simulink model "IcingFTISystem_simulator_rev0"  (R2021b)
settings: Solver=ode23tb  StartTime=0.0  StopTime=360  MaxStep=0.1  RelTol=1e-6
libraries: simulink x2
settings Model: Creator=julia  LastModifiedBy=julia
settings SolverCC: InitialStep=0.1

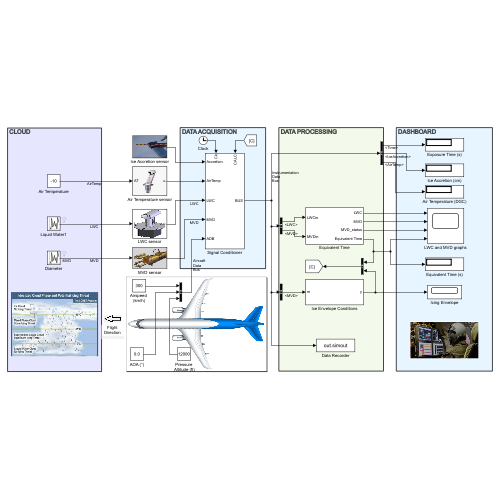
[thumbnail: Simulink's stored preview of the top-level diagram]
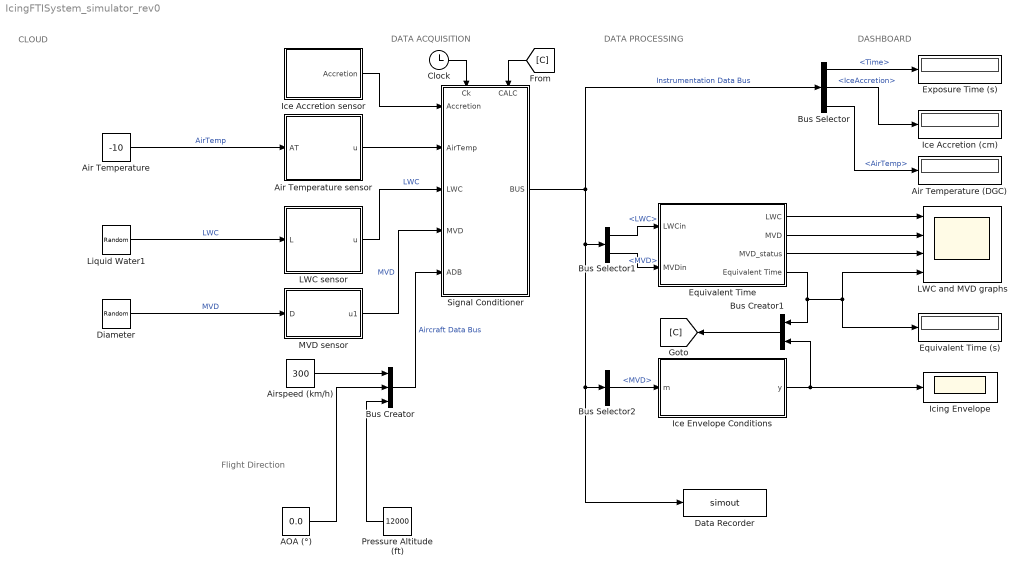
== system IcingFTISystem_simulator_rev0 ==
  note: Flight
      | Direction
  note: CLOUD
  note: DATA ACQUISITION
  note: DASHBOARD
  note: DATA PROCESSING
  AOA (°) : Constant  Value=0.0
  Air Temperature : Constant  Value=-10
  Air Temperature (DGC) : Display
  Air Temperature sensor : Subsystem
      mask Display: image('C:\Users\julia\Desktop\MEstrado\Sensores Manuais\Imagens 2022\TemperatureSensor1.jpg'); % Use "Edit Image" on toolstrip to change.
  Airspeed (km/h) : Constant  Value=300
  Bus Creator : BusCreator  Inputs=3
  Bus Creator1 : BusCreator  Inputs=2
  Bus Selector : BusSelector  OutputSignals=Time,IceAccretion,AirTemp
  Bus Selector1 : BusSelector  OutputSignals=LWC,MVD
  Bus Selector2 : BusSelector  OutputSignals=MVD
  Clock : Clock
  Data Recorder : ToWorkspace  VariableName=simout  SampleTime=1
      settings: Save2DSignal=2-D array (concatenate along first dimension)
  Diameter : UniformRandomNumber  Minimum=0  Maximum=51  SampleTime=0.5
  Equivalent Time : Subsystem
  Equivalent Time (s) : Display
  Exposure Time (s) : Display
  Ice Accretion (cm) : Display
  Ice Accretion sensor : Subsystem
      mask Display: image('C:\Users\julia\Desktop\MEstrado\Sensores Manuais\Imagens 2022\IceAccretion.jpg'); % Use "Edit Image" on toolstrip to change.
  Ice Envelope Conditions : Subsystem
  Icing Envelope : Scope
  LWC and MVD graphs : Scope  NumInputPorts=4
  LWC sensor : Subsystem
      mask Display: image('C:\Users\julia\Desktop\MEstrado\Sensores Manuais\Imagens 2022\MultielementProbe.jpg'); % Use "Edit Image" on toolstrip to change.
  Liquid Water1 : UniformRandomNumber  Minimum=0.1  Maximum=0.7  SampleTime=0.1
  MVD sensor : Subsystem
      mask Display: image('C:\Users\julia\Desktop\MEstrado\Sensores Manuais\Imagens 2022\MVDprobe.jpg'); % Use "Edit Image" on toolstrip to change.
  Pressure Altitude (ft) : Constant  Value=12000
  Signal Conditioner : Subsystem
      settings: PortSchema="{\"entries\":[{\"content\":{\"sides\":[{\"content\":{\"connectorIds\":[\"In1\",\"In2\",\"In3\",\"In4\",\"In5\"]},\"type\":\"ConnectorPlacement.EquallySpacedRectSide\",\"uuid\":\"37654887-8b06-403a-8d28-0bf4ed0ace53\"},{\"content\":{\"connectorIds\":[\"Out1\"],\"side\":\"RIGHT\"},\"type\":\"ConnectorPlacement.EquallySpacedRectSide\",\"uuid\":\"06b92d83-e4db-41b5-b404-488771456c30\"},{\"content\":{\"connectorIds\":[\"In6\",\"In7\"],\"side\":\"TOP\"},\"type\":\"ConnectorPlacement.EquallySpacedRectSide\",\"uuid\":\"374586bc-ca22-4ce3-837a-6311d85410d9\"}]},\"type\":\"ConnectorPlacement.EquallySpacedConnector\",\"uuid\":\"530a5a3a-e051-406d-b434-132ac86c67f6\"}],\"packageUris\":[\"http://schema.mathworks.com/mf0/Connector/R2020b\"],\"version\":\"1.0\"}"
  wires:
  LWC sensor/1(u) -> Signal Conditioner/3(LWC)  "LWC"
  MVD sensor/1(u1) -> Signal Conditioner/4(MVD)  "MVD"
  Equivalent Time/1(LWC) -> LWC and MVD graphs/1
  Equivalent Time/2(MVD) -> LWC and MVD graphs/2
  Equivalent Time/3(MVD_status) -> LWC and MVD graphs/3
  Air Temperature sensor/1(u) -> Signal Conditioner/2(AirTemp)
  Ice Accretion sensor/1(Accretion) -> Signal Conditioner/1(Accretion)
  Air Temperature/1 -> Air Temperature sensor/1(AT)  "AirTemp"
  Diameter/1 -> MVD sensor/1(D)  "MVD"
  Liquid Water1/1 -> LWC sensor/1(L)  "LWC"
  Clock/1 -> Signal Conditioner/6(Ck)
  Signal Conditioner/1(BUS) -> Data Recorder/1, Bus Selector2/1, Bus Selector1/1, Bus Selector/1  "Instrumentation Data Bus"
  Bus Selector/1 -> Exposure Time (s)/1  "<Time>"
  Bus Selector/2 -> Ice Accretion (cm)/1  "<IceAccretion>"
  Bus Selector/3 -> Air Temperature (DGC)/1  "<AirTemp>"
  Bus Selector1/1 -> Equivalent Time/1(LWCin)  "<LWC>"
  Bus Selector1/2 -> Equivalent Time/2(MVDin)  "<MVD>"
  Equivalent Time/4(Equivalent Time) -> Bus Creator1/1, LWC and MVD graphs/4, Equivalent Time (s)/1
  Ice Envelope Conditions/1(y) -> Bus Creator1/2, Icing Envelope/1
  Bus Selector2/1 -> Ice Envelope Conditions/1(m)  "<MVD>"
  Airspeed (km/h)/1 -> Bus Creator/1
  AOA (°)/1 -> Bus Creator/2
  Pressure Altitude (ft)/1 -> Bus Creator/3
  Bus Creator/1 -> Signal Conditioner/5(ADB)  "Aircraft Data Bus"
  Bus Creator1/1 -> [C]
  [C] -> Signal Conditioner/7(CALC)

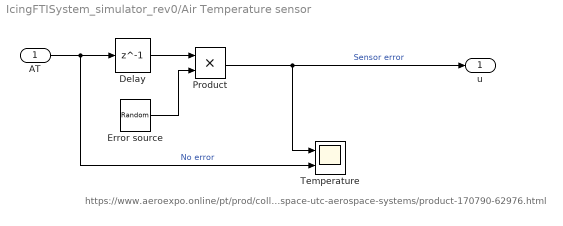
== system IcingFTISystem_simulator_rev0/Air Temperature sensor ==
  note: https://www.aeroexpo.online/pt/prod/collins-aerospace-utc-aerospace-systems/product-170790-62976.html
  AT : Inport
  Delay : Delay  DelayLength=1
  Error source : UniformRandomNumber  Minimum=0.95  Maximum=1.1  Seed=1  SampleTime=0.1
  Product : Product
  Temperature : Scope  NumInputPorts=2
  u : Outport
  wires:
  Product/1 -> u/1, Temperature/1  "Sensor error"
  AT/1 -> Delay/1, Temperature/2  "No error"
  Error source/1 -> Product/2
  Delay/1 -> Product/1

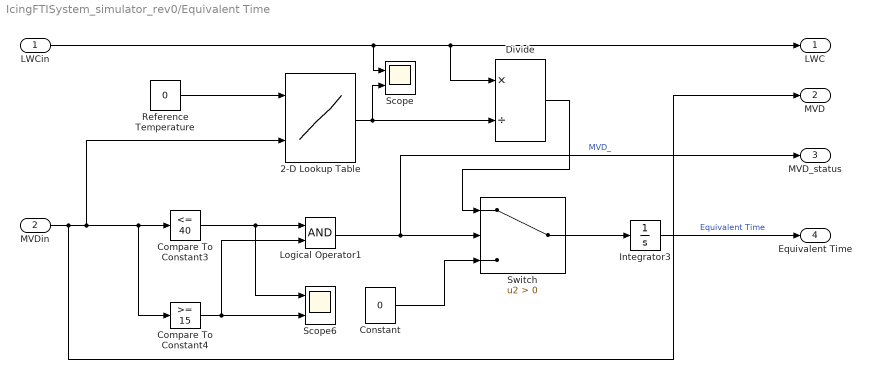
== system IcingFTISystem_simulator_rev0/Equivalent Time ==
  LWCin : Inport
  MVDin : Inport  Port=2
  2-D Lookup Table : Lookup_n-D  BreakpointsForDimension1=[0 10 20 30]  BreakpointsForDimension2=[15 25 30 40]  Table=[0.8 0.5 0.375 0.155; 0.59 0.3 0.22 0.1; 0.3 0.15 0.11 0.6; 0.2 0.1 0.1 0.04]  InternalRulePriority=Speed  RndMeth=Simplest  InputSameDT=on
      settings: InputPortMap=u0,u1
  Compare To Constant3 : simulink/Logic and Bit Operations/Compare To Constant  relop=<=  const=40  OutDataTypeStr=uint8
  Compare To Constant4 : simulink/Logic and Bit Operations/Compare To Constant  relop=>=  const=15  OutDataTypeStr=uint8
  Constant : Constant  Value=0
  Divide : Product  Inputs=*/
  Integrator3 : Integrator
  Logical Operator1 : Logic  AllPortsSameDT=off  OutDataTypeStr=boolean
  Reference Temperature : Constant  Value=0
  Scope : Scope  NumInputPorts=2
  Scope6 : Scope  NumInputPorts=2
  Switch : Switch  Criteria=u2 > Threshold
  LWC : Outport
  MVD : Outport  Port=2
  MVD_status : Outport  Port=3
  Equivalent Time : Outport  Port=4
  wires:
  Compare To Constant3/1 -> Scope6/1, Logical Operator1/1
  Integrator3/1 -> Equivalent Time/1  "Equivalent Time"
  Compare To Constant4/1 -> Logical Operator1/2, Scope6/2
  MVDin/1 -> MVD/1, 2-D Lookup Table/2, Compare To Constant3/1, Compare To Constant4/1
  Reference Temperature/1 -> 2-D Lookup Table/1
  Logical Operator1/1 -> MVD_status/1, Switch/2  "MVD_"
  Constant/1 -> Switch/3
  2-D Lookup Table/1 -> Scope/2, Divide/2
  LWCin/1 -> Scope/1, LWC/1, Divide/1
  Divide/1 -> Switch/1
  Switch/1 -> Integrator3/1

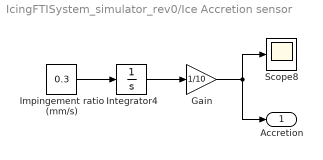
== system IcingFTISystem_simulator_rev0/Ice Accretion sensor ==
  Gain : Gain  Gain=1/10
  Impingement ratio (mm/s) : Constant  Value=0.3
  Integrator4 : Integrator
  Scope8 : Scope
  Accretion : Outport
  wires:
  Gain/1 -> Accretion/1, Scope8/1
  Integrator4/1 -> Gain/1
  Impingement ratio (mm/s)/1 -> Integrator4/1

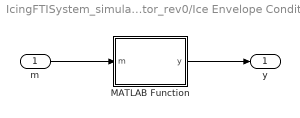
== system IcingFTISystem_simulator_rev0/Ice Envelope Conditions ==
  m : Inport
  MATLAB Function : MATLAB Function  TreatAsAtomicUnit=on
  y : Outport
  wires:
  m/1 -> MATLAB Function/1(m)
  MATLAB Function/1(y) -> y/1

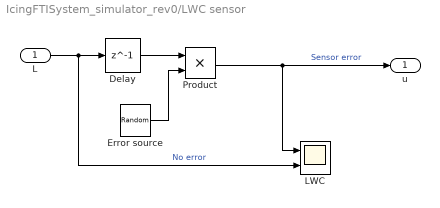
== system IcingFTISystem_simulator_rev0/LWC sensor ==
  L : Inport
  Delay : Delay  DelayLength=1
  Error source : UniformRandomNumber  Minimum=0.9  Maximum=1.1  Seed=1  SampleTime=0.1
  LWC : Scope  NumInputPorts=2
  Product : Product
  u : Outport
  wires:
  Product/1 -> u/1, LWC/1  "Sensor error"
  L/1 -> Delay/1, LWC/2  "No error"
  Error source/1 -> Product/2
  Delay/1 -> Product/1

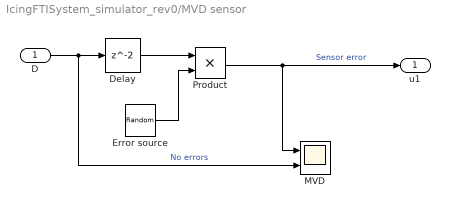
== system IcingFTISystem_simulator_rev0/MVD sensor ==
  D : Inport
  Delay : Delay
  Error source : UniformRandomNumber  Minimum=0.9  Maximum=1.1  Seed=1  SampleTime=0.1
  MVD : Scope  NumInputPorts=2
  Product : Product
  u1 : Outport
  wires:
  Product/1 -> MVD/1, u1/1  "Sensor error"
  D/1 -> Delay/1, MVD/2  "No errors"
  Error source/1 -> Product/2
  Delay/1 -> Product/1

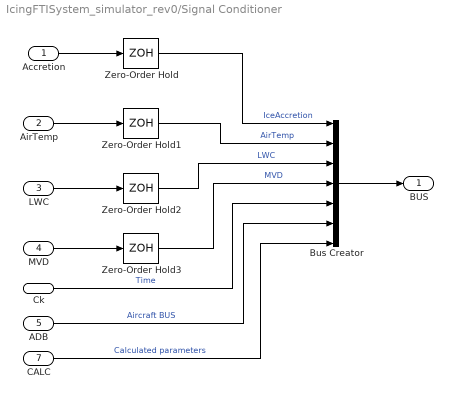
== system IcingFTISystem_simulator_rev0/Signal Conditioner ==
  Accretion : Inport
  AirTemp : Inport  Port=2
  LWC : Inport  Port=3
  MVD : Inport  Port=4
  ADB : Inport  Port=5
  Ck : Inport  Port=6
  CALC : Inport  Port=7
  Bus Creator : BusCreator  Inputs=7
  Zero-Order Hold{,1..3} (4 alike) : ZeroOrderHold  SampleTime=0.1
  BUS : Outport
  wires:
  Accretion/1 -> Zero-Order Hold/1
  Zero-Order Hold/1 -> Bus Creator/1  "IceAccretion"
  Zero-Order Hold1/1 -> Bus Creator/2  "AirTemp"
  Zero-Order Hold2/1 -> Bus Creator/3  "LWC"
  Zero-Order Hold3/1 -> Bus Creator/4  "MVD"
  MVD/1 -> Zero-Order Hold3/1
  Bus Creator/1 -> BUS/1
  Ck/1 -> Bus Creator/5  "Time"
  AirTemp/1 -> Zero-Order Hold1/1
  LWC/1 -> Zero-Order Hold2/1
  ADB/1 -> Bus Creator/6  "Aircraft BUS"
  CALC/1 -> Bus Creator/7  "Calculated parameters"

== matlab function IcingFTISystem_simulator_rev0/Ice Envelope Conditions/MATLAB Function ==
  data: m input; y output
function y = fcn(m)

if (m > 500)
    y = 3;
    elseif (m > 100) && (m < 500)
    y = 2;
elseif (m > 15) && (m < 40)
        y = 1;
else y = 0;
end
